simulink model "WindowDiscriminator"  (R2020a)
settings: Solver=VariableStepAuto  StartTime=0  StopTime=10  RelTol=1e-3
model workspace (MAT data in the model file):
  dac_stop_max = 3
  threshold = [-50; -300]
  win_start = [0; 0]
  win_stop = [3; 3]
values from neighbouring files (symbols this model uses):
  DAC_enable1 = 1    [run_WindowDiscriminator.m]
  DAC_enable2 = 1    [run_WindowDiscriminator.m]
  DAC_enable3 = 1    [run_WindowDiscriminator.m]
  DAC_enable4 = 1    [run_WindowDiscriminator.m]
  DAC_enable5 = 0    [run_WindowDiscriminator.m]
  DAC_enable6 = 0    [run_WindowDiscriminator.m]
  DAC_enable7 = 0    [run_WindowDiscriminator.m]
  DAC_enable8 = 0    [run_WindowDiscriminator.m]
  DAC_type1 = 0    [run_WindowDiscriminator.m]
  DAC_type2 = 1    [run_WindowDiscriminator.m]
  DAC_type3 = 1    [run_WindowDiscriminator.m]
  DAC_type4 = 1    [run_WindowDiscriminator.m]
  DAC_type5 = 0    [run_WindowDiscriminator.m]
  DAC_type6 = 0    [run_WindowDiscriminator.m]
  DAC_type7 = 0    [run_WindowDiscriminator.m]
  DAC_type8 = 0    [run_WindowDiscriminator.m]
  fs = 30000    [run_AdaptiveThreshold.m]    (also in run_AdaptiveThresholdLocalMaxima.m; run_HardThreshold.m; run_HardThresholdLocalMaxima.m; run_LocalMaxima_AdaptiveThreshold.m)
  refractory = 10^-3    (= 0.001)    [run_AdaptiveThreshold.m]    (also in run_AdaptiveThresholdLocalMaxima.m; run_HardThreshold.m; run_HardThresholdLocalMaxima.m; run_LocalMaxima_AdaptiveThreshold.m)
  start1 = 0    [run_WindowDiscriminator.m]
  start2 = 1    [run_WindowDiscriminator.m]
  start3 = 4    [run_WindowDiscriminator.m]
  start4 = 3    [run_WindowDiscriminator.m]
  start5 = 3    [run_WindowDiscriminator.m]
  start6 = 3    [run_WindowDiscriminator.m]
  start7 = 3    [run_WindowDiscriminator.m]
  start8 = 3    [run_WindowDiscriminator.m]
  stop1 = 1    [run_WindowDiscriminator.m]
  stop2 = 6    [run_WindowDiscriminator.m]
  stop3 = 11    [run_WindowDiscriminator.m]
  stop4 = 15    [run_WindowDiscriminator.m]
  stop5 = 2    [run_WindowDiscriminator.m]
  stop6 = 2    [run_WindowDiscriminator.m]
  stop7 = 2    [run_WindowDiscriminator.m]
  stop8 = 2    [run_WindowDiscriminator.m]
  th1 = [-39.975]    [run_WindowDiscriminator.m]
  th2 = [-148.98]    [run_WindowDiscriminator.m]
  th3 = [-24.96]    [run_WindowDiscriminator.m]
  th4 = [13.065]    [run_WindowDiscriminator.m]
  th5 = [-11]    [run_WindowDiscriminator.m]
  th6 = [-11]    [run_WindowDiscriminator.m]
  th7 = [-11]    [run_WindowDiscriminator.m]
  th8 = [-11]    [run_WindowDiscriminator.m]
libraries: simulink x21, dspfdesign x2, dspswit3 x1, hdlsllib x1
settings Model: Creator=stefanobuccelli  LastModifiedBy=diflo
settings DataIOCC: ReturnWorkspaceOutputs=off
settings DebuggingCC: ArithmeticOperatorsInVariantConditions=warning
settings SFSimCC: SimUseLocalCustomCode=off  CustomCodeUndefinedFunction=UseInterfaceOnly
settings RTWCC: RTWUseLocalCustomCode=off

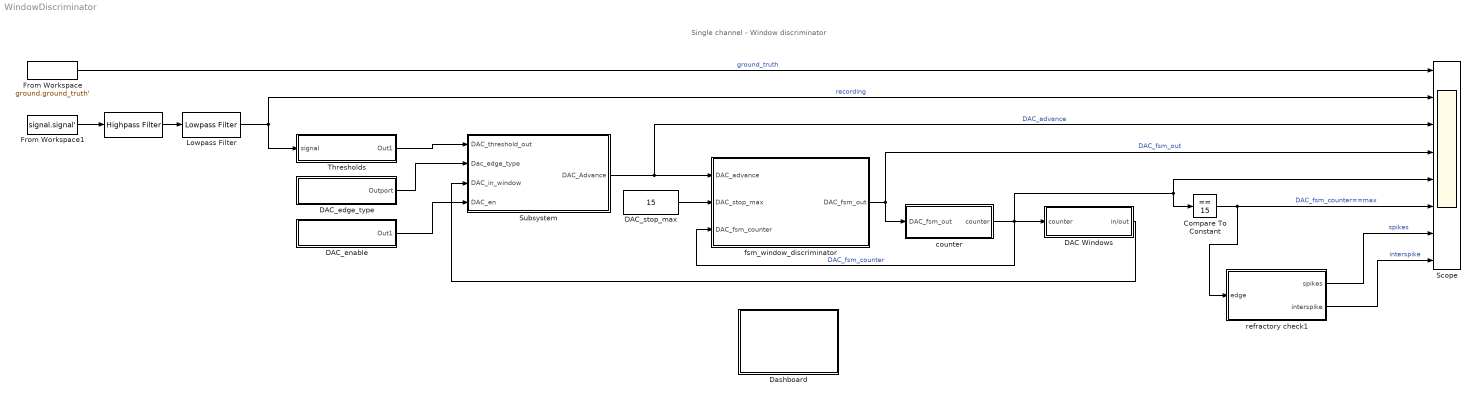
== system WindowDiscriminator ==
  note: Single channel - Window discriminator
  " " : dspfdesign/Highpass Filter  FilterType=IIR  DesignForMinimumOrder=on  FilterOrder=50  StopbandFrequency=1  PassbandFrequency=300  StopbandAttenuation=80  PassbandRipple=0.1  InheritSampleRate=off  SampleRate=fs  SimulateUsing=Interpreted execution  roundingMode=Floor  coeffsDataTypeStr=fixdt(1,16)
  Compare To Constant : simulink/Logic and Bit Operations/Compare To Constant  relop===  const=15  OutDataTypeStr=boolean
  DAC Windows : Subsystem
  DAC_edge_type : Subsystem
  DAC_enable : Subsystem
  DAC_stop_max : Constant  Value=15  OutDataTypeStr=double
  Dashboard : Subsystem
  From Workspace : FromWorkspace  VariableName=ground.ground_truth'  SampleTime=1/fs
  From Workspace1 : FromWorkspace  VariableName=signal.signal'  SampleTime=1/fs
  Lowpass Filter : dspfdesign/Lowpass Filter  FilterType=IIR  DesignForMinimumOrder=on  FilterOrder=3  PassbandFrequency=3500  StopbandFrequency=8500  PassbandRipple=0.1  StopbandAttenuation=80  InheritSampleRate=off  SampleRate=fs  SimulateUsing=Interpreted execution  roundingMode=Floor  coeffsDataTypeStr=fixdt(1,16)
  Scope : Scope  NumInputPorts=8
  Subsystem : Subsystem
  Thresholds : Subsystem
  counter : Subsystem
  fsm_window_discriminator : Stateflow chart  TreatAsAtomicUnit=on
  refractory check1 : Subsystem
  wires:
  fsm_window_discriminator/1(DAC_fsm_out) -> counter/1(DAC_fsm_out), Scope/4  "DAC_fsm_out"
  Subsystem/1(DAC_Advance) -> Scope/3, fsm_window_discriminator/1(DAC_advance)  "DAC_advance"
  DAC_edge_type/1(Outport) -> Subsystem/2(Dac_edge_type)
  DAC_stop_max/1 -> fsm_window_discriminator/2(DAC_stop_max)
  DAC Windows/1(in/out) -> Subsystem/3(DAC_in_window)
  Thresholds/1(Out1) -> Subsystem/1(DAC_threshold_out)
  DAC_enable/1(Out1) -> Subsystem/4(DAC_en)
  counter/1(counter) -> DAC Windows/1(counter), fsm_window_discriminator/3(DAC_fsm_counter), Scope/5, Compare To Constant/1  "DAC_fsm_counter"
  Compare To Constant/1 -> refractory check1/1(" edge "), Scope/6  "DAC_fsm_counter==max"
  refractory check1/1(spikes) -> Scope/7  "spikes"
  refractory check1/2(interspike) -> Scope/8  "interspike"
  Lowpass Filter/1 -> Scope/2, Thresholds/1(signal)  "recording"
  From Workspace/1 -> Scope/1  "ground_truth"
  " "/1 -> Lowpass Filter/1
  From Workspace1/1 -> " "/1

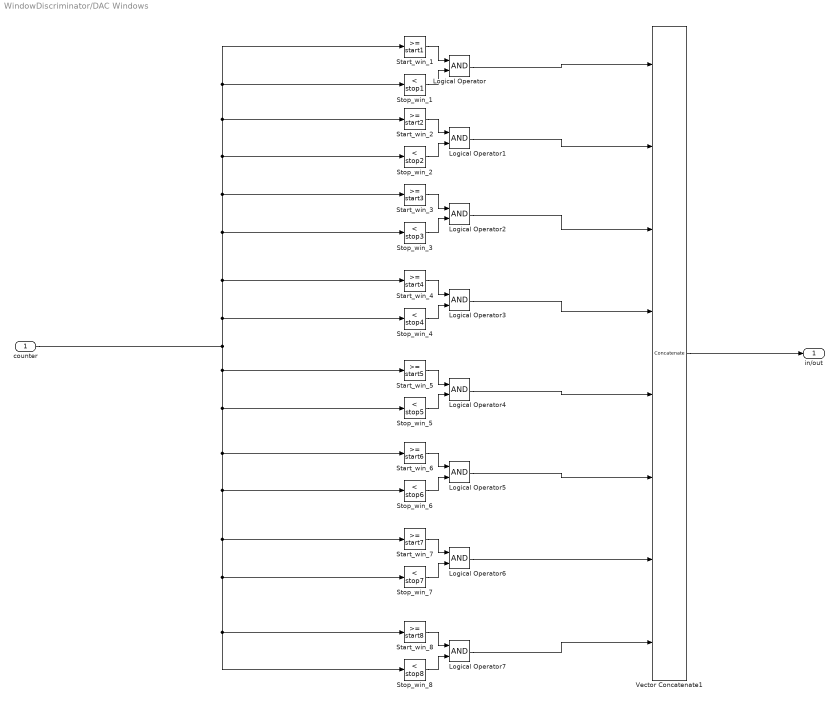
== system WindowDiscriminator/DAC Windows ==
  counter : Inport
  Logical Operator{,1..7} (8 alike) : Logic  AllPortsSameDT=off  OutDataTypeStr=boolean
  Start_win_1 : simulink/Logic and Bit Operations/Compare To Constant  relop=>=  const=start1  OutDataTypeStr=boolean
  Start_win_2 : simulink/Logic and Bit Operations/Compare To Constant  relop=>=  const=start2  OutDataTypeStr=boolean
  Start_win_3 : simulink/Logic and Bit Operations/Compare To Constant  relop=>=  const=start3  OutDataTypeStr=boolean
  Start_win_4 : simulink/Logic and Bit Operations/Compare To Constant  relop=>=  const=start4  OutDataTypeStr=boolean
  Start_win_5 : simulink/Logic and Bit Operations/Compare To Constant  relop=>=  const=start5  OutDataTypeStr=boolean
  Start_win_6 : simulink/Logic and Bit Operations/Compare To Constant  relop=>=  const=start6  OutDataTypeStr=boolean
  Start_win_7 : simulink/Logic and Bit Operations/Compare To Constant  relop=>=  const=start7  OutDataTypeStr=boolean
  Start_win_8 : simulink/Logic and Bit Operations/Compare To Constant  relop=>=  const=start8  OutDataTypeStr=boolean
  Stop_win_1 : simulink/Logic and Bit Operations/Compare To Constant  relop=<  const=stop1  OutDataTypeStr=boolean
  Stop_win_2 : simulink/Logic and Bit Operations/Compare To Constant  relop=<  const=stop2  OutDataTypeStr=boolean
  Stop_win_3 : simulink/Logic and Bit Operations/Compare To Constant  relop=<  const=stop3  OutDataTypeStr=boolean
  Stop_win_4 : simulink/Logic and Bit Operations/Compare To Constant  relop=<  const=stop4  OutDataTypeStr=boolean
  Stop_win_5 : simulink/Logic and Bit Operations/Compare To Constant  relop=<  const=stop5  OutDataTypeStr=boolean
  Stop_win_6 : simulink/Logic and Bit Operations/Compare To Constant  relop=<  const=stop6  OutDataTypeStr=boolean
  Stop_win_7 : simulink/Logic and Bit Operations/Compare To Constant  relop=<  const=stop7  OutDataTypeStr=boolean
  Stop_win_8 : simulink/Logic and Bit Operations/Compare To Constant  relop=<  const=stop8  OutDataTypeStr=boolean
  Vector Concatenate1 : Concatenate  NumInputs=8
  in/out : Outport  VectorParamsAs1DForOutWhenUnconnected=off
  wires:
  Vector Concatenate1/1 -> in/out/1
  Stop_win_1/1 -> Logical Operator/2
  Start_win_1/1 -> Logical Operator/1
  Logical Operator/1 -> Vector Concatenate1/1
  Logical Operator1/1 -> Vector Concatenate1/2
  Stop_win_2/1 -> Logical Operator1/2
  Start_win_2/1 -> Logical Operator1/1
  Stop_win_3/1 -> Logical Operator2/2
  Start_win_3/1 -> Logical Operator2/1
  Logical Operator2/1 -> Vector Concatenate1/3
  Start_win_4/1 -> Logical Operator3/1
  Stop_win_4/1 -> Logical Operator3/2
  Logical Operator3/1 -> Vector Concatenate1/4
  Stop_win_5/1 -> Logical Operator4/2
  Start_win_5/1 -> Logical Operator4/1
  Logical Operator4/1 -> Vector Concatenate1/5
  Start_win_6/1 -> Logical Operator5/1
  Logical Operator5/1 -> Vector Concatenate1/6
  Stop_win_6/1 -> Logical Operator5/2
  Stop_win_7/1 -> Logical Operator6/2
  Start_win_7/1 -> Logical Operator6/1
  Logical Operator6/1 -> Vector Concatenate1/7
  Stop_win_8/1 -> Logical Operator7/2
  Start_win_8/1 -> Logical Operator7/1
  Logical Operator7/1 -> Vector Concatenate1/8
  counter/1 -> Stop_win_5/1, Start_win_6/1, Stop_win_6/1, Start_win_7/1, Stop_win_7/1, Start_win_8/1, Stop_win_8/1, Start_win_5/1, Stop_win_4/1, Start_win_4/1, Stop_win_3/1, Start_win_3/1, Stop_win_2/1, Start_win_2/1, Stop_win_1/1, Start_win_1/1

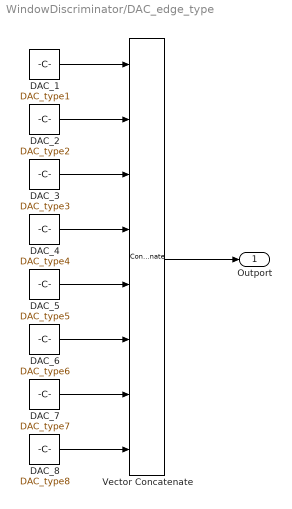
== system WindowDiscriminator/DAC_edge_type ==
  DAC_1 : Constant  Value=DAC_type1
  DAC_2 : Constant  Value=DAC_type2
  DAC_3 : Constant  Value=DAC_type3
  DAC_4 : Constant  Value=DAC_type4
  DAC_5 : Constant  Value=DAC_type5
  DAC_6 : Constant  Value=DAC_type6
  DAC_7 : Constant  Value=DAC_type7
  DAC_8 : Constant  Value=DAC_type8
  Vector Concatenate : Concatenate  NumInputs=8
  Outport : Outport  VectorParamsAs1DForOutWhenUnconnected=off
  wires:
  DAC_7/1 -> Vector Concatenate/7
  DAC_6/1 -> Vector Concatenate/6
  DAC_1/1 -> Vector Concatenate/1
  Vector Concatenate/1 -> Outport/1
  DAC_5/1 -> Vector Concatenate/5
  DAC_8/1 -> Vector Concatenate/8
  DAC_4/1 -> Vector Concatenate/4
  DAC_3/1 -> Vector Concatenate/3
  DAC_2/1 -> Vector Concatenate/2

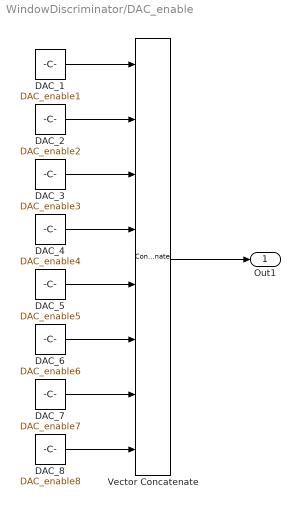
== system WindowDiscriminator/DAC_enable ==
  DAC_1 : Constant  Value=DAC_enable1
  DAC_2 : Constant  Value=DAC_enable2
  DAC_3 : Constant  Value=DAC_enable3
  DAC_4 : Constant  Value=DAC_enable4
  DAC_5 : Constant  Value=DAC_enable5
  DAC_6 : Constant  Value=DAC_enable6
  DAC_7 : Constant  Value=DAC_enable7
  DAC_8 : Constant  Value=DAC_enable8
  Vector Concatenate : Concatenate  NumInputs=8
  Out1 : Outport  VectorParamsAs1DForOutWhenUnconnected=off
  wires:
  DAC_1/1 -> Vector Concatenate/1
  DAC_4/1 -> Vector Concatenate/4
  DAC_2/1 -> Vector Concatenate/2
  DAC_8/1 -> Vector Concatenate/8
  Vector Concatenate/1 -> Out1/1
  DAC_3/1 -> Vector Concatenate/3
  DAC_7/1 -> Vector Concatenate/7
  DAC_5/1 -> Vector Concatenate/5
  DAC_6/1 -> Vector Concatenate/6

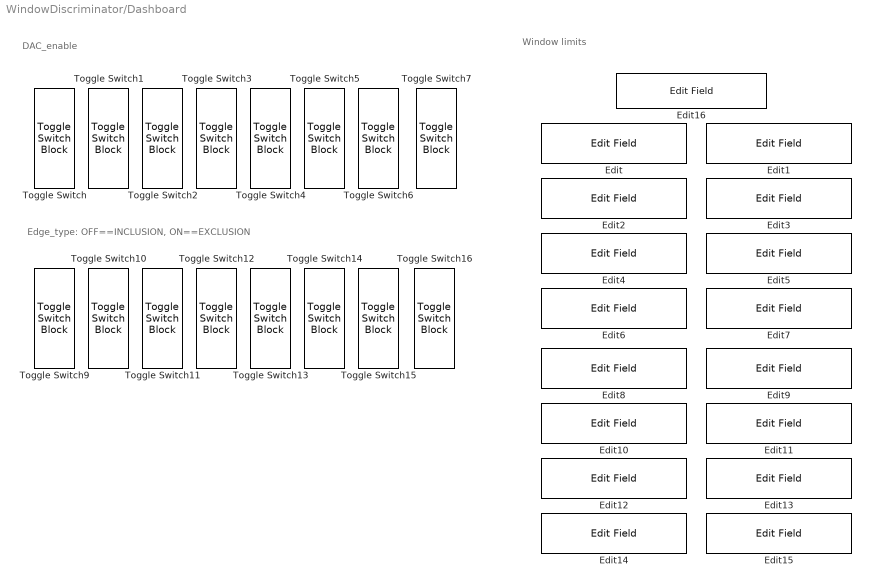
== system WindowDiscriminator/Dashboard ==
  note: Window limits
  note: Edge_type: OFF==INCLUSION, ON==EXCLUSION
  note: DAC_enable
  Edit{,1..16} (17 alike) : EditField  Alignment=Center
  Toggle Switch{,1..7,9..16} (16 alike) : ToggleSwitchBlock
      settings: Values={{'Off', 'On'}, [0 1]}

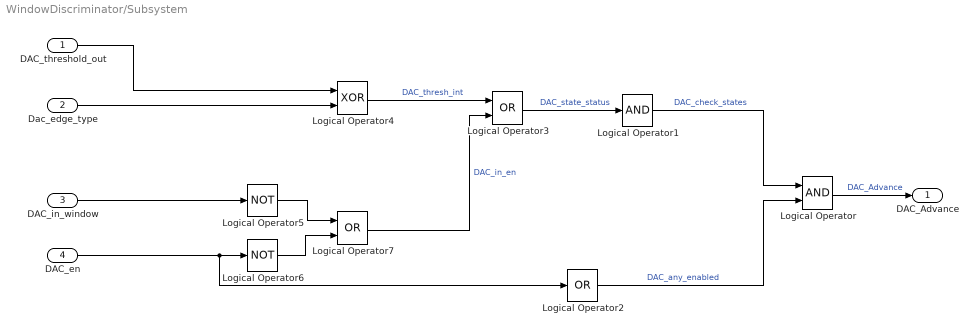
== system WindowDiscriminator/Subsystem ==
  DAC_threshold_out : Inport
  Dac_edge_type : Inport  Port=2
  DAC_in_window : Inport  Port=3
  DAC_en : Inport  Port=4
  Logical Operator : Logic  AllPortsSameDT=off  OutDataTypeStr=boolean
  Logical Operator1 : Logic  Inputs=1  AllPortsSameDT=off  OutDataTypeStr=boolean
  Logical Operator2 : Logic  Operator=OR  Inputs=1  AllPortsSameDT=off  OutDataTypeStr=boolean
  Logical Operator3 : Logic  Operator=OR  AllPortsSameDT=off  OutDataTypeStr=boolean
  Logical Operator4 : Logic  Operator=XOR  AllPortsSameDT=off  OutDataTypeStr=boolean
  Logical Operator5 : Logic  Operator=NOT  Inputs=1  AllPortsSameDT=off  OutDataTypeStr=boolean
  Logical Operator6 : Logic  Operator=NOT  Inputs=1  AllPortsSameDT=off  OutDataTypeStr=boolean
  Logical Operator7 : Logic  Operator=OR  AllPortsSameDT=off  OutDataTypeStr=boolean
  DAC_Advance : Outport  VectorParamsAs1DForOutWhenUnconnected=off
  wires:
  Logical Operator/1 -> DAC_Advance/1  "DAC_Advance"
  Logical Operator2/1 -> Logical Operator/2  "DAC_any_enabled"
  Logical Operator1/1 -> Logical Operator/1  "DAC_check_states"
  Logical Operator4/1 -> Logical Operator3/1  "DAC_thresh_int"
  Logical Operator5/1 -> Logical Operator7/1
  DAC_threshold_out/1 -> Logical Operator4/1
  DAC_en/1 -> Logical Operator2/1, Logical Operator6/1
  Logical Operator3/1 -> Logical Operator1/1  "DAC_state_status"
  Logical Operator6/1 -> Logical Operator7/2
  Logical Operator7/1 -> Logical Operator3/2  "DAC_in_en"
  Dac_edge_type/1 -> Logical Operator4/2
  DAC_in_window/1 -> Logical Operator5/1

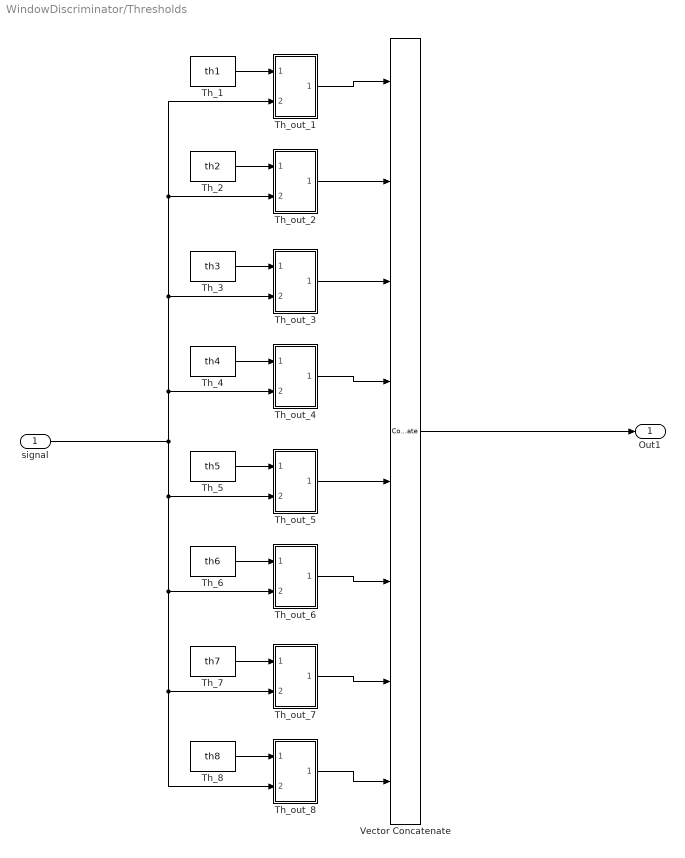
== system WindowDiscriminator/Thresholds ==
  signal : Inport
  Th_1 : Constant  Value=th1  OutDataTypeStr=double  LockScale=on
  Th_2 : Constant  Value=th2  OutDataTypeStr=double  LockScale=on
  Th_3 : Constant  Value=th3  OutDataTypeStr=double  LockScale=on
  Th_4 : Constant  Value=th4  OutDataTypeStr=double  LockScale=on
  Th_5 : Constant  Value=th5  OutDataTypeStr=double  LockScale=on
  Th_6 : Constant  Value=th6  OutDataTypeStr=double  LockScale=on
  Th_7 : Constant  Value=th7  OutDataTypeStr=double  LockScale=on
  Th_8 : Constant  Value=th8  OutDataTypeStr=double  LockScale=on
  Th_out_1 : Subsystem
  Th_out_2 : Subsystem
  Th_out_3 : Subsystem
  Th_out_4 : Subsystem
  Th_out_5 : Subsystem
  Th_out_6 : Subsystem
  Th_out_7 : Subsystem
  Th_out_8 : Subsystem
  Vector Concatenate : Concatenate  NumInputs=8
  Out1 : Outport  VectorParamsAs1DForOutWhenUnconnected=off
  wires:
  Vector Concatenate/1 -> Out1/1
  Th_1/1 -> Th_out_1/1(In1)
  Th_2/1 -> Th_out_2/1(In1)
  Th_4/1 -> Th_out_4/1(In1)
  Th_3/1 -> Th_out_3/1(In1)
  Th_6/1 -> Th_out_6/1(In1)
  Th_7/1 -> Th_out_7/1(In1)
  Th_8/1 -> Th_out_8/1(In1)
  Th_5/1 -> Th_out_5/1(In1)
  Th_out_2/1(Out1) -> Vector Concatenate/2
  Th_out_3/1(Out1) -> Vector Concatenate/3
  Th_out_4/1(Out1) -> Vector Concatenate/4
  Th_out_5/1(Out1) -> Vector Concatenate/5
  Th_out_6/1(Out1) -> Vector Concatenate/6
  Th_out_8/1(Out1) -> Vector Concatenate/8
  Th_out_7/1(Out1) -> Vector Concatenate/7
  signal/1 -> Th_out_4/2(In2), Th_out_1/2(In2), Th_out_2/2(In2), Th_out_3/2(In2), Th_out_8/2(In2), Th_out_7/2(In2), Th_out_6/2(In2), Th_out_5/2(In2)
  Th_out_1/1(Out1) -> Vector Concatenate/1

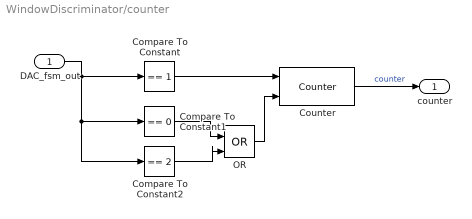
== system WindowDiscriminator/counter ==
  DAC_fsm_out : Inport
  Compare To Constant : simulink/Logic and Bit Operations/Compare To Constant  relop===  const=1  OutDataTypeStr=boolean
  Compare To Constant1 : simulink/Logic and Bit Operations/Compare To Constant  relop===  const=0  OutDataTypeStr=boolean
  Compare To Constant2 : simulink/Logic and Bit Operations/Compare To Constant  relop===  const=2  OutDataTypeStr=boolean
  Counter : dspswit3/Counter  Direction=Up  CountEvent=Non-zero sample  CounterSize=User defined  MaxCount=255  InitialCount=0  Output=Count  HitValue=32  ResetInput=on  SamplesPerFrame=1  Ts=1  CntDtype=double  HitDtype=Logical
  OR : Logic  Operator=OR  IconShape=distinctive  AllPortsSameDT=off  OutDataTypeStr=boolean
  counter : Outport  VectorParamsAs1DForOutWhenUnconnected=off
  wires:
  Counter/1 -> counter/1  "counter"
  Compare To Constant2/1 -> OR/2
  Compare To Constant/1 -> Counter/1
  Compare To Constant1/1 -> OR/1
  OR/1 -> Counter/2
  DAC_fsm_out/1 -> Compare To Constant2/1, Compare To Constant1/1, Compare To Constant/1

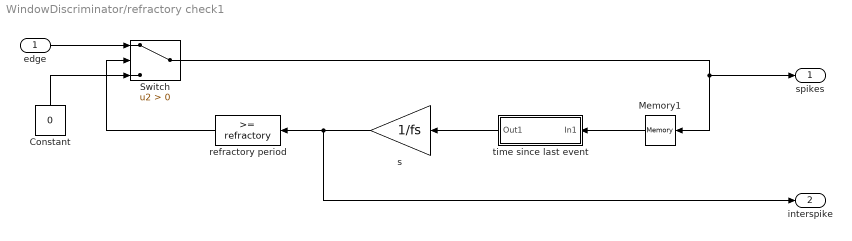
== system WindowDiscriminator/refractory check1 ==
  " edge " : Inport
  Constant : Constant  Value=0
  Memory1 : Memory  InheritSampleTime=on
  Switch : Switch  Criteria=u2 > Threshold
  refractory period : simulink/Logic and Bit Operations/Compare To Constant  relop=>=  const=refractory  OutDataTypeStr=boolean
  s : Gain  Gain=1/fs  ParamDataTypeStr=double
  time since last event : Subsystem
  spikes : Outport
  interspike : Outport  Port=2
  wires:
  " edge "/1 -> Switch/1
  Memory1/1 -> time since last event/1(In1)
  time since last event/1(Out1) -> s/1
  Constant/1 -> Switch/3
  s/1 -> refractory period/1, interspike/1
  Switch/1 -> spikes/1, Memory1/1
  refractory period/1 -> Switch/2

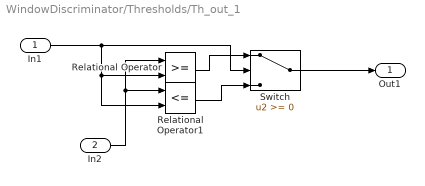
== system WindowDiscriminator/Thresholds/Th_out_1 ==
  In1 : Inport
  In2 : Inport  Port=2
  Relational Operator : RelationalOperator  OutDataTypeStr=boolean  RndMeth=Simplest
  Relational Operator1 : RelationalOperator  Operator=<=  OutDataTypeStr=boolean  RndMeth=Simplest
  Switch : Switch
  Out1 : Outport  VectorParamsAs1DForOutWhenUnconnected=off
  wires:
  Relational Operator/1 -> Switch/1
  Relational Operator1/1 -> Switch/3
  In1/1 -> Switch/2, Relational Operator1/2, Relational Operator/2
  Switch/1 -> Out1/1
  In2/1 -> Relational Operator/1, Relational Operator1/1

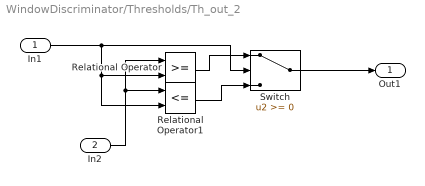
== system WindowDiscriminator/Thresholds/Th_out_2 ==
  In1 : Inport
  In2 : Inport  Port=2
  Relational Operator : RelationalOperator  OutDataTypeStr=boolean  RndMeth=Simplest
  Relational Operator1 : RelationalOperator  Operator=<=  OutDataTypeStr=boolean  RndMeth=Simplest
  Switch : Switch
  Out1 : Outport  VectorParamsAs1DForOutWhenUnconnected=off
  wires:
  Relational Operator/1 -> Switch/1
  Relational Operator1/1 -> Switch/3
  In1/1 -> Switch/2, Relational Operator1/2, Relational Operator/2
  Switch/1 -> Out1/1
  In2/1 -> Relational Operator/1, Relational Operator1/1

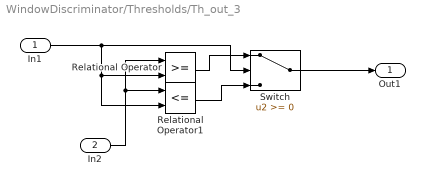
== system WindowDiscriminator/Thresholds/Th_out_3 ==
  In1 : Inport
  In2 : Inport  Port=2
  Relational Operator : RelationalOperator  OutDataTypeStr=boolean  RndMeth=Simplest
  Relational Operator1 : RelationalOperator  Operator=<=  OutDataTypeStr=boolean  RndMeth=Simplest
  Switch : Switch
  Out1 : Outport  VectorParamsAs1DForOutWhenUnconnected=off
  wires:
  Relational Operator/1 -> Switch/1
  Relational Operator1/1 -> Switch/3
  In1/1 -> Switch/2, Relational Operator1/2, Relational Operator/2
  Switch/1 -> Out1/1
  In2/1 -> Relational Operator/1, Relational Operator1/1

== system WindowDiscriminator/Thresholds/Th_out_4 ==
  In1 : Inport
  In2 : Inport  Port=2
  Relational Operator : RelationalOperator  OutDataTypeStr=boolean  RndMeth=Simplest
  Relational Operator1 : RelationalOperator  Operator=<=  OutDataTypeStr=boolean  RndMeth=Simplest
  Switch : Switch
  Out1 : Outport  VectorParamsAs1DForOutWhenUnconnected=off
  wires:
  Relational Operator/1 -> Switch/1
  Relational Operator1/1 -> Switch/3
  In1/1 -> Switch/2, Relational Operator1/2, Relational Operator/2
  Switch/1 -> Out1/1
  In2/1 -> Relational Operator/1, Relational Operator1/1

== system WindowDiscriminator/Thresholds/Th_out_5 ==
  In1 : Inport
  In2 : Inport  Port=2
  Relational Operator : RelationalOperator  OutDataTypeStr=boolean  RndMeth=Simplest
  Relational Operator1 : RelationalOperator  Operator=<=  OutDataTypeStr=boolean  RndMeth=Simplest
  Switch : Switch
  Out1 : Outport  VectorParamsAs1DForOutWhenUnconnected=off
  wires:
  Relational Operator/1 -> Switch/1
  Relational Operator1/1 -> Switch/3
  In1/1 -> Switch/2, Relational Operator1/2, Relational Operator/2
  Switch/1 -> Out1/1
  In2/1 -> Relational Operator/1, Relational Operator1/1

== system WindowDiscriminator/Thresholds/Th_out_6 ==
  In1 : Inport
  In2 : Inport  Port=2
  Relational Operator : RelationalOperator  OutDataTypeStr=boolean  RndMeth=Simplest
  Relational Operator1 : RelationalOperator  Operator=<=  OutDataTypeStr=boolean  RndMeth=Simplest
  Switch : Switch
  Out1 : Outport  VectorParamsAs1DForOutWhenUnconnected=off
  wires:
  Relational Operator/1 -> Switch/1
  Relational Operator1/1 -> Switch/3
  In1/1 -> Switch/2, Relational Operator1/2, Relational Operator/2
  Switch/1 -> Out1/1
  In2/1 -> Relational Operator/1, Relational Operator1/1

== system WindowDiscriminator/Thresholds/Th_out_7 ==
  In1 : Inport
  In2 : Inport  Port=2
  Relational Operator : RelationalOperator  OutDataTypeStr=boolean  RndMeth=Simplest
  Relational Operator1 : RelationalOperator  Operator=<=  OutDataTypeStr=boolean  RndMeth=Simplest
  Switch : Switch
  Out1 : Outport  VectorParamsAs1DForOutWhenUnconnected=off
  wires:
  Relational Operator/1 -> Switch/1
  Relational Operator1/1 -> Switch/3
  In1/1 -> Switch/2, Relational Operator1/2, Relational Operator/2
  Switch/1 -> Out1/1
  In2/1 -> Relational Operator/1, Relational Operator1/1

== system WindowDiscriminator/Thresholds/Th_out_8 ==
  In1 : Inport
  In2 : Inport  Port=2
  Relational Operator : RelationalOperator  OutDataTypeStr=boolean  RndMeth=Simplest
  Relational Operator1 : RelationalOperator  Operator=<=  OutDataTypeStr=boolean  RndMeth=Simplest
  Switch : Switch
  Out1 : Outport  VectorParamsAs1DForOutWhenUnconnected=off
  wires:
  Relational Operator/1 -> Switch/1
  Relational Operator1/1 -> Switch/3
  In1/1 -> Switch/2, Relational Operator1/2, Relational Operator/2
  Switch/1 -> Out1/1
  In2/1 -> Relational Operator/1, Relational Operator1/1

== system WindowDiscriminator/refractory check1/time since last event ==
  In1 : Inport
  HDL Counter : hdlsllib/Sources/HDL Counter  CountType=Free running  CountInit=1  CountStep=1  CountMax=25  CountFromType=Initial value  CountFrom=1  CountResetPort=on  CountLoadPort=off  CountEnbPort=off  CountDirPort=off  CountDataType=Unsigned  CountWordLen=32  CountFracLen=0  CountSampTime=1
  Out1 : Outport
  wires:
  In1/1 -> HDL Counter/1
  HDL Counter/1 -> Out1/1

== stateflow chart WindowDiscriminator/fsm_window_discriminator ==
  settings: stateMachineType=MOORE_MACHINE  executeAtInitialization=1
  state IDLE
    DAC_fsm_out=0
  state TRACK
    DAC_fsm_out=1
  state STIM
    DAC_fsm_out=2
  (default) -> IDLE
  STIM -> IDLE
  TRACK -> IDLE [order 2] : [~DAC_advance]
  IDLE -> TRACK : [DAC_advance]
  TRACK -> TRACK [order 3] : [DAC_fsm_counter~=DAC_stop_max]
  TRACK -> STIM [order 1] : [DAC_fsm_counter==DAC_stop_max]
  data: DAC_advance input; DAC_fsm_out output double =0; DAC_stop_max input; DAC_fsm_counter input double =0
